simulink model "q_loop"  (R2019a)
settings: Solver=ode45  StartTime=0.0  StopTime=10.0  MaxStep=0.01  RelTol=1e-3
values from neighbouring files (symbols this model uses):
  A = SS_long.A    [PlacePoles.m]
  B = SS_long.B(:, 2)    [PlacePoles.m]
  Ka = F(1)    [PlacePoles.m]
  Kq = F(2)    [PlacePoles.m]
undefined symbols (not defined in the file or in its folder): C_pp, D_pp
libraries: cstblocks x2, simulink_extras x1
settings Model: Creator=tblaha  LastModifiedBy=tblaha
settings SolverCC: SolverOrder=5

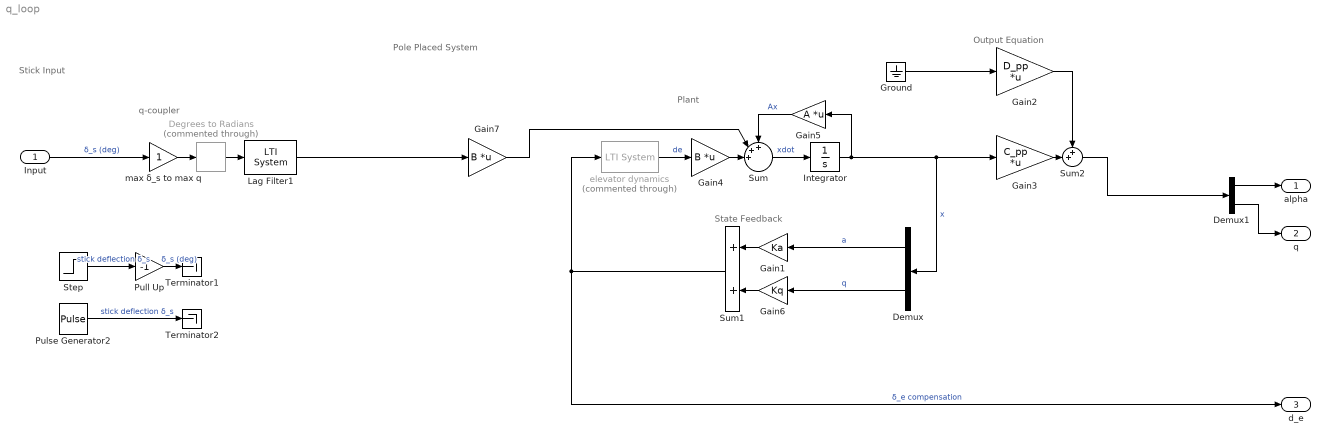
== system q_loop ==
  note: Plant
  note: State Feedback
  note: Output Equation
  note: Stick Input
  note: Pole Placed System
  note: q-coupler
  Input : Inport
  Degrees to Radians : simulink_extras/Transformations/Degrees to Radians  Commented=through
  Demux : Demux  Outputs=2
  Demux1 : Demux  Outputs=2
  Gain1 : Gain  Gain=Ka
  Gain2 : Gain  Gain=D_pp  Multiplication=Matrix(K*u)
  Gain3 : Gain  Gain=C_pp  Multiplication=Matrix(K*u)
  Gain4 : Gain  Gain=B  Multiplication=Matrix(K*u)
  Gain5 : Gain  Gain=A  Multiplication=Matrix(K*u)
  Gain6 : Gain  Gain=Kq
  Gain7 : Gain  Gain=B  Multiplication=Matrix(K*u)
  Ground : Ground
  Integrator : Integrator  InitialCondition=[0 0]  ContinuousStateAttributes=['alpha', 'q']
  Lag Filter1 : cstblocks/LTI System  sys=LL_filt  IC=[]
  Pull Up : Gain  Gain=-1
  Pulse Generator2 : DiscretePulseGenerator  PulseType=Time based  Period=10  PulseWidth=60  PhaseDelay=1
  Step : Step  After=10  SampleTime=0
  Sum : Sum  Inputs=+++||
  Sum1 : Sum
  Sum2 : Sum  Inputs=++|
  Terminator1 : Terminator
  Terminator2 : Terminator
  elevator dynamics : cstblocks/LTI System  Commented=through  sys=H_servo  IC=[]
  max δ_s to max q : Gain
  alpha : Outport
  q : Outport  Port=2
  d_e : Outport  Port=3
  wires:
  Gain2/1 -> Sum2/1
  Sum2/1 -> Demux1/1
  Demux/1 -> Gain1/1  "a"
  Demux/2 -> Gain6/1  "q"
  Gain1/1 -> Sum1/1
  Gain6/1 -> Sum1/2
  Gain3/1 -> Sum2/2
  Lag Filter1/1 -> Gain7/1
  Integrator/1 -> Gain3/1, Demux/1, Gain5/1  "x"
  Sum1/1 -> d_e/1, elevator dynamics/1  "δ_e compensation"
  elevator dynamics/1 -> Gain4/1  "de"
  Gain4/1 -> Sum/3
  Gain5/1 -> Sum/1  "Ax"
  Sum/1 -> Integrator/1  "xdot"
  Input/1 -> max δ_s to max q/1  "δ_s (deg)"
  Gain7/1 -> Sum/2
  Degrees to Radians/1 -> Lag Filter1/1
  max δ_s to max q/1 -> Degrees to Radians/1
  Pulse Generator2/1 -> Terminator2/1  "stick deflection δ_s"
  Step/1 -> Pull Up/1  "stick deflection δ_s"
  Pull Up/1 -> Terminator1/1  "δ_s (deg)"
  Ground/1 -> Gain2/1
  Demux1/1 -> alpha/1
  Demux1/2 -> q/1
